simulink model "RRR_ADct"  (R2022a)
settings: Solver=VariableStepAuto  StartTime=0.0  StopTime=1500  RelTol=1e-6
undefined symbols (not defined in the file): B_ADct, DiscIntNeverNeededParam, dq0, Kp_CTad, Kv_CTad, Levenberg, m1, m2, m3, Marquardt, p0, P_ADct, param, Pi, Pi_hat0_ADct, q0, r0, r1, r2, R_ADct, slow
libraries: simulink x2, robotmaniplib x1
settings Model: PauseTimes=0.14  Creator=Mathew  LastModifiedBy=Marco
settings SolverCC: ZeroCrossControl=DisableAll  ODENIntegrationMethod=ode1be
settings DebuggingCC: AlgebraicLoopMsg=none  UnconnectedInputMsg=warning  UnconnectedOutputMsg=warning  UnconnectedLineMsg=warning  SFMachineParentedDataDiag=warning
settings SFSimCC: CustomCodeUndefinedFunction=UseInterfaceOnly
settings RTWCC: DLArmComputeVersion=19.05

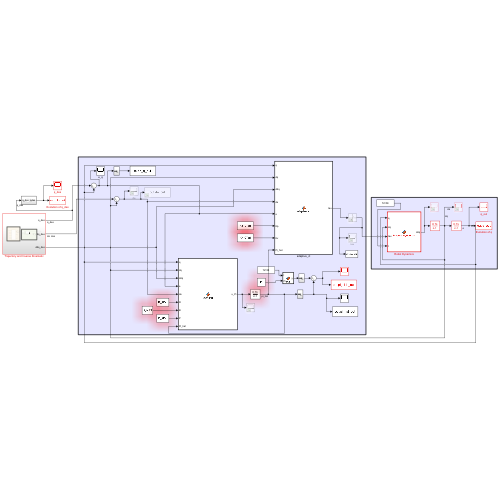
[thumbnail: Simulink's stored preview of the top-level diagram]
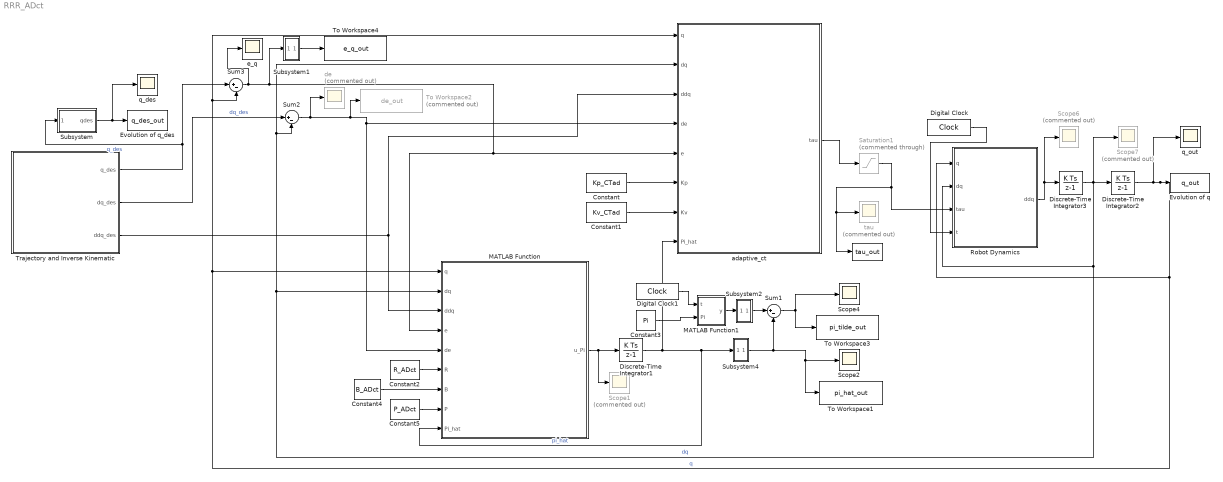
== system RRR_ADct ==
  "         " : ToWorkspace  VariableName=tau_out  SaveFormat=Timeseries  SampleTime=-1
  Constant : Constant  Value=Kp_CTad
  Constant1 : Constant  Value=Kv_CTad
  Constant2 : Constant  Value=R_ADct
  Constant3 : Constant  Value=Pi
  Constant4 : Constant  Value=B_ADct
  Constant5 : Constant  Value=P_ADct
  Digital Clock : DigitalClock  SampleTime=0.01
  Digital Clock1 : DigitalClock  SampleTime=0.01
  Discrete-Time Integrator1 : DiscreteIntegrator  InitialCondition=Pi_hat0_ADct  SampleTime=-1  ICPrevOutput=DiscIntNeverNeededParam  ICPrevScaledInput=DiscIntNeverNeededParam
  Discrete-Time Integrator2 : DiscreteIntegrator  InitialCondition=q0  SampleTime=-1  ICPrevOutput=DiscIntNeverNeededParam  ICPrevScaledInput=DiscIntNeverNeededParam
  Discrete-Time Integrator3 : DiscreteIntegrator  InitialCondition=dq0  SampleTime=-1  ICPrevOutput=DiscIntNeverNeededParam  ICPrevScaledInput=DiscIntNeverNeededParam
  Evolution of q : ToWorkspace  VariableName=q_out  SaveFormat=Timeseries  SampleTime=-1
  Evolution of q_des : ToWorkspace  VariableName=q_des_out  SaveFormat=Timeseries  SampleTime=-1
  MATLAB Function : MATLAB Function  TreatAsAtomicUnit=on
  MATLAB Function1 : MATLAB Function  TreatAsAtomicUnit=on
  Robot Dynamics : MATLAB Function  TreatAsAtomicUnit=on
  Saturation1 : Saturate  Commented=through  UpperLimit=100  LowerLimit=-100
  Scope1 : Scope  Commented=on
  Scope2 : Scope
  Scope4 : Scope
  Scope6 : Scope  Commented=on
  Scope7 : Scope  Commented=on
  Subsystem : Subsystem
  Subsystem1 : Subsystem
  Subsystem2 : Subsystem
  Subsystem4 : Subsystem
  Sum1 : Sum  Inputs=|+-
  Sum2 : Sum  Inputs=|+-
  Sum3 : Sum  Inputs=|+-
  To Workspace1 : ToWorkspace  VariableName=pi_hat_out  SaveFormat=Timeseries  SampleTime=-1
  To Workspace2 : ToWorkspace  Commented=on  VariableName=de_out  SaveFormat=Timeseries  SampleTime=-1
  To Workspace3 : ToWorkspace  VariableName=pi_tilde_out  SaveFormat=Timeseries  SampleTime=-1
  To Workspace4 : ToWorkspace  VariableName=e_q_out  SaveFormat=Timeseries  SampleTime=-1
  Trajectory and Inverse Kinematic : Subsystem
  adaptive_ct : MATLAB Function  TreatAsAtomicUnit=on
  de : Scope  Commented=on
  e_q : Scope
  q_des : Scope
  q_out : Scope
  tau : Scope  Commented=on
  wires:
  Constant/1 -> adaptive_ct/6(Kp)
  adaptive_ct/1(tau) -> Saturation1/1
  MATLAB Function/1(u_Pi) -> Discrete-Time Integrator1/1, Scope1/1
  Sum1/1 -> Scope4/1, To Workspace3/1
  Constant3/1 -> MATLAB Function1/2(Pi)
  Discrete-Time Integrator1/1 -> adaptive_ct/8(Pi_hat), Subsystem4/1(eq), MATLAB Function/9(Pi_hat)  "pi_hat"
  Constant2/1 -> MATLAB Function/6(R)
  Constant1/1 -> adaptive_ct/7(Kv)
  Sum2/1 -> To Workspace2/1, adaptive_ct/4(de), MATLAB Function/5(de), de/1
  Sum3/1 -> Subsystem1/1(eq), MATLAB Function/4(e), adaptive_ct/5(e), e_q/1
  Constant4/1 -> MATLAB Function/7(B)
  Constant5/1 -> MATLAB Function/8(P)
  Robot Dynamics/1(ddq) -> Discrete-Time Integrator3/1, Scope6/1
  Discrete-Time Integrator2/1 -> Robot Dynamics/1(q), Sum3/2, adaptive_ct/1(q), MATLAB Function/1(q), Evolution of q/1, q_out/1  "q"
  Discrete-Time Integrator3/1 -> Robot Dynamics/2(dq), adaptive_ct/2(dq), Sum2/2, MATLAB Function/2(dq), Scope7/1, Discrete-Time Integrator2/1  "dq"
  Saturation1/1 -> Robot Dynamics/3(tau), "         "/1, tau/1
  Subsystem/1(qdes) -> q_des/1, Evolution of q_des/1
  Trajectory and Inverse Kinematic/1(q_des) -> Sum3/1, Subsystem/1(q_des)  "q_des"
  Trajectory and Inverse Kinematic/2(dq_des) -> Sum2/1  "dq_des"
  Trajectory and Inverse Kinematic/3(ddq_des) -> adaptive_ct/3(ddq), MATLAB Function/3(ddq)
  Digital Clock/1 -> Robot Dynamics/4(t)
  Subsystem1/1(eq_) -> To Workspace4/1
  Subsystem4/1(eq_) -> Scope2/1, To Workspace1/1, Sum1/2
  MATLAB Function1/1(y) -> Subsystem2/1(eq)
  Digital Clock1/1 -> MATLAB Function1/1(t)
  Subsystem2/1(eq_) -> Sum1/1

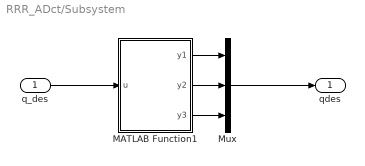
== system RRR_ADct/Subsystem ==
  q_des : Inport
  MATLAB Function1 : MATLAB Function  TreatAsAtomicUnit=on
  Mux : Mux  Inputs=3
  qdes : Outport
  wires:
  MATLAB Function1/1(y1) -> Mux/1
  Mux/1 -> qdes/1
  q_des/1 -> MATLAB Function1/1(u)
  MATLAB Function1/2(y2) -> Mux/2
  MATLAB Function1/3(y3) -> Mux/3

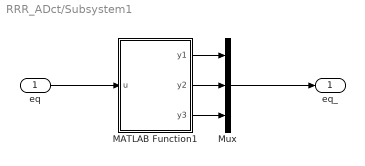
== system RRR_ADct/Subsystem1 ==
  eq : Inport
  MATLAB Function1 : MATLAB Function  TreatAsAtomicUnit=on
  Mux : Mux  Inputs=3
  eq_ : Outport
  wires:
  MATLAB Function1/1(y1) -> Mux/1
  Mux/1 -> eq_/1
  eq/1 -> MATLAB Function1/1(u)
  MATLAB Function1/2(y2) -> Mux/2
  MATLAB Function1/3(y3) -> Mux/3

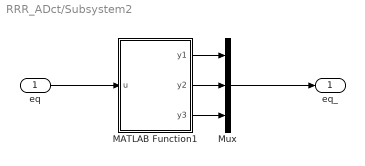
== system RRR_ADct/Subsystem2 ==
  eq : Inport
  MATLAB Function1 : MATLAB Function  TreatAsAtomicUnit=on
  Mux : Mux  Inputs=3
  eq_ : Outport
  wires:
  MATLAB Function1/1(y1) -> Mux/1
  Mux/1 -> eq_/1
  eq/1 -> MATLAB Function1/1(u)
  MATLAB Function1/2(y2) -> Mux/2
  MATLAB Function1/3(y3) -> Mux/3

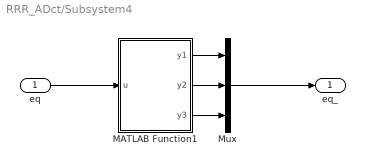
== system RRR_ADct/Subsystem4 ==
  eq : Inport
  MATLAB Function1 : MATLAB Function  TreatAsAtomicUnit=on
  Mux : Mux  Inputs=3
  eq_ : Outport
  wires:
  MATLAB Function1/3(y3) -> Mux/3
  MATLAB Function1/2(y2) -> Mux/2
  eq/1 -> MATLAB Function1/1(u)
  Mux/1 -> eq_/1
  MATLAB Function1/1(y1) -> Mux/1

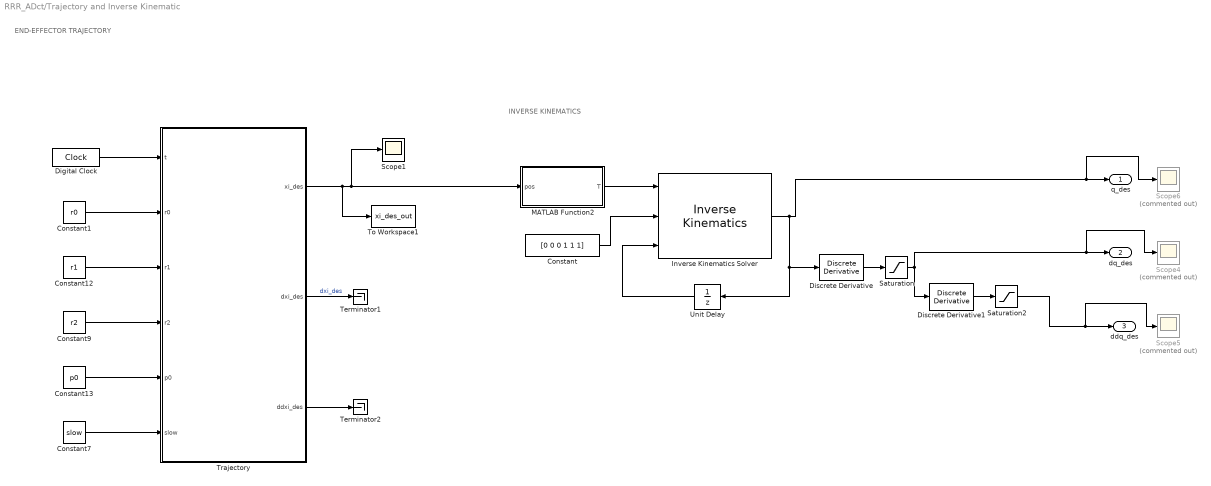
== system RRR_ADct/Trajectory and Inverse Kinematic ==
  note: END-EFFECTOR TRAJECTORY
  note: INVERSE KINEMATICS
  Constant : Constant  Value=[0 0 0 1 1 1]
  Constant1 : Constant  Value=r0
  Constant12 : Constant  Value=r1
  Constant13 : Constant  Value=p0
  Constant7 : Constant  Value=slow
  Constant9 : Constant  Value=r2
  Digital Clock : DigitalClock  SampleTime=0.01
  Discrete Derivative : simulink/Discrete/Discrete Derivative  gainval=1  ICPrevScaledInput=q0  OutMin=-1  OutMax=1  OutDataType=fixdt(1, 16)  OutScaling=2^-10  DoSatur=on
  Discrete Derivative1 : simulink/Discrete/Discrete Derivative  gainval=1.0  ICPrevScaledInput=ddq0  OutMin=[]  OutMax=[]  OutDataType=fixdt(1, 16)  OutScaling=2^-10  DoSatur=off
  Inverse Kinematics Solver : robotmaniplib/Inverse Kinematics  RigidBodyTree=ur10e_bis  EndEffector=body3  ShowInfo=off  SolverName=Levenberg-Marquardt  EnforceJointLimits=on  MaxIterations=1500  MaxTime=10  GradientTolerance=1e-7  SolutionTolerance=1e-5  StepTolerance=1e-14  ErrorChangeTolerance=1e-8  UseErrorDamping=on  DampingBias=0.0025  SimulateUsing=Interpreted execution
  MATLAB Function2 : MATLAB Function  TreatAsAtomicUnit=on
  Saturation : Saturate
  Saturation2 : Saturate  UpperLimit=0.1  LowerLimit=-0.1
  Scope1 : Scope
  Scope4 : Scope  Commented=on
  Scope5 : Scope  Commented=on
  Scope6 : Scope  Commented=on
  Terminator1 : Terminator
  Terminator2 : Terminator
  To Workspace1 : ToWorkspace  VariableName=xi_des_out  SaveFormat=Timeseries  SampleTime=-1
  Trajectory : MATLAB Function  TreatAsAtomicUnit=on
  Unit Delay : UnitDelay  SampleTime=-1  HasFrameUpgradeWarning=on
  q_des : Outport  VectorParamsAs1DForOutWhenUnconnected=off
  dq_des : Outport  Port=2  VectorParamsAs1DForOutWhenUnconnected=off
  ddq_des : Outport  Port=3  VectorParamsAs1DForOutWhenUnconnected=off
  wires:
  Trajectory/1(xi_des) -> Scope1/1, MATLAB Function2/1(pos), To Workspace1/1
  Constant13/1 -> Trajectory/5(p0)
  Constant7/1 -> Trajectory/6(slow)
  Constant9/1 -> Trajectory/4(r2)
  Constant12/1 -> Trajectory/3(r1)
  Trajectory/3(ddxi_des) -> Terminator2/1
  Inverse Kinematics Solver/1 -> Unit Delay/1, Discrete Derivative/1, Scope6/1, q_des/1
  Constant/1 -> Inverse Kinematics Solver/2
  MATLAB Function2/1(T) -> Inverse Kinematics Solver/1
  Unit Delay/1 -> Inverse Kinematics Solver/3
  Digital Clock/1 -> Trajectory/1(t)
  Trajectory/2(dxi_des) -> Terminator1/1  "dxi_des"
  Discrete Derivative/1 -> Saturation/1
  Discrete Derivative1/1 -> Saturation2/1
  Saturation/1 -> Discrete Derivative1/1, Scope4/1, dq_des/1
  Saturation2/1 -> Scope5/1, ddq_des/1
  Constant1/1 -> Trajectory/2(r0)

== matlab function RRR_ADct/Subsystem2/MATLAB Function1 ==
  data: u input; y1 output; y2 output; y3 output
function [y1,y2,y3] = fcn(u)

y1 = squeeze(u(1));
y2 = squeeze(u(2));
y3 = squeeze(u(3));

== matlab function RRR_ADct/Subsystem4/MATLAB Function1 ==
  data: u input; y1 output; y2 output; y3 output
function [y1,y2,y3] = fcn(u)

y1 = squeeze(u(1));
y2 = squeeze(u(2));
y3 = squeeze(u(3));

== matlab function RRR_ADct/Trajectory and Inverse Kinematic/MATLAB Function2 ==
  data: pos input; T output
function T = homogeneus_transf(pos)
    
    T=eye(4);
    
    T = [  eye(3),     [pos(1);pos(2);pos(3) ];
         0 0 0              1           ]; 

end

== matlab function RRR_ADct/MATLAB Function ==
  data: q input; u_Pi output; dq input; ddq input; e input; de input; R input; B input; P input; Pi_hat input; param parameter
function u_Pi = updating(q, dq, ddq, e, de, R, B, P, Pi_hat, param)
  
    g = 9.81;
    
    Y = Y_fun(g,param,ddq,dq,q);
    
    M_hat = B_3r(param,Pi_hat(1),Pi_hat(2),Pi_hat(3),q);
    
    x = [e; de];
    
    u_Pi = - pinv(R) * Y' * (pinv(M_hat,1e-3))' * B' * P * x;

end

== matlab function RRR_ADct/Subsystem1/MATLAB Function1 ==
  data: u input; y1 output; y2 output; y3 output
function [y1,y2,y3] = fcn(u)

y1 = squeeze(u(1));
y2 = squeeze(u(2));
y3 = squeeze(u(3));

== matlab function RRR_ADct/Robot Dynamics ==
  data: q input; dq input; tau input; t input; ddq output; m1 parameter; m2 parameter; m3 parameter; param parameter
function ddq = inverse_dynamics(q, dq, tau, t, m1, m2, m3, param)
    
    g = 9.81;

    if t > 200
        m2 = m2 + 1;
    end

    % Get dynamic matrices
    M = B_3r(param,m1,m2,m3,q);
    C = C_3r(param,m1,m2,m3,q,dq);
    G = G_3r(g,param,m1,m2,m3,q);
    
    ddq = pinv(M)*(tau - C*dq - G);

end

== matlab function RRR_ADct/Subsystem/MATLAB Function1 ==
  data: u input; y1 output; y2 output; y3 output
function [y1,y2,y3] = fcn(u)

y1 = squeeze(u(1));
y2 = squeeze(u(2));
y3 = squeeze(u(3));

== matlab function RRR_ADct/adaptive_ct ==
  data: q input; dq input; ddq input; tau output; de input; e input; Kp input; Kv input; Pi_hat input; param parameter
function tau = adaptive_ct(q, dq, ddq, de, e, Kp, Kv, Pi_hat, param)

    g = 9.81;
    
    Y = Y_fun(g,param,ddq,dq,q);
    
    % Control law
    tau = Y*Pi_hat + Kv*de + Kp*e;

end

== matlab function RRR_ADct/Trajectory and Inverse Kinematic/Trajectory ==
  data: t input; r0 input; xi_des output; r1 input; r2 input; p0 input; slow input; dxi_des output; ddxi_des output
function [xi_des, dxi_des, ddxi_des] = trajectory(t,r0,r1,r2,p0,slow)

    k=slow;
    
    xi_des =   [r0*sin(t/(2*k))       ; r1*sin(t/k)     ; r2*cos(t/k)     ] + p0;
    dxi_des =  [r0/2/k*cos(t/(2*k))   ; r1/k*cos(t/k)   ; -r2/k*sin(t/k)  ];
    ddxi_des = [-r0/4/k/k*sin(t/(2*k)); -r1/k/k*sin(t/k); -r2/k/k*cos(t/k)];

end

== matlab function RRR_ADct/MATLAB Function1 ==
  data: t input; Pi input; y output
function y = fcn(t,Pi)

    if t > 200
        Pi(2) = Pi(2) + 1;
    end

    y = Pi;

end
